simulink model "PlantaMalhaExterna"  (R2021a)
settings: Solver=VariableStepAuto  StartTime=0.0  StopTime=10.0  RelTol=1e-3
libraries: pid_lib x1
settings Model: Creator=lucas  LastModifiedBy=lucas

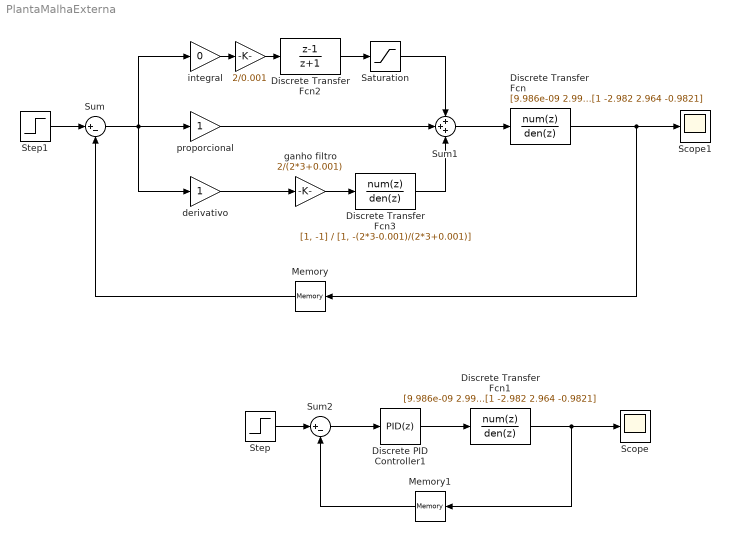
== system PlantaMalhaExterna ==
  " " : Gain  Gain=2/0.001
  Discrete Transfer Fcn : DiscreteTransferFcn  Numerator=[9.986e-09 2.996e-08 2.996e-08 9.986e-09]  Denominator=[1 -2.982 2.964 -0.9821]  SampleTime=0.001
  Discrete Transfer Fcn1 : DiscreteTransferFcn  Numerator=[9.986e-09 2.996e-08 2.996e-08 9.986e-09]  Denominator=[1 -2.982 2.964 -0.9821]  SampleTime=0.001
  Discrete Transfer Fcn2 : DiscreteTransferFcn  Numerator=[1, -1]  Denominator=[1, 1]
  Discrete Transfer Fcn3 : DiscreteTransferFcn  Numerator=[1, -1]  Denominator=[1, -(2*3-0.001)/(2*3+0.001)]  SampleTime=0.001
  Discrete PID Controller1 : pid_lib/PID Controller  Controller=PID  Form=Parallel  TimeDomain=Discrete-time  UseExternalTs=off  SampleTime=0.001  IntegratorMethod=Forward Euler  FilterMethod=Forward Euler  ControllerParametersSource=internal  P=200  I=0  D=8  UseFilter=on  N=1.824  TunerSelectOption=Transfer Function Based (PID Tuner App)  InitialConditionSource=internal  InitialConditionForIntegrator=0  InitialConditionForFilter=0  DifferentiatorICPrevScaledInput=0  ExternalReset=none  TrackingMode=off  Kt=1  LimitOutput=off  SatLimitsSource=internal  UpperSaturationLimit=inf  LowerSaturationLimit=-inf  LinearizeAsGain=off  AntiWindupMode=none  Kb=1  POutMin=[]  POutMax=[]  IOutMin=[]  IOutMax=[]  DOutMin=[]  DOutMax=[]  NOutMin=[]  NOutMax=[]  SumOutMin=[]  SumOutMax=[]  SaturationOutMin=[]  SaturationOutMax=[]  PParamMin=[]  PParamMax=[]  IParamMin=[]  IParamMax=[]  DParamMin=[]  DParamMax=[]  NParamMin=[]  NParamMax=[]  KbParamMin=[]  KbParamMax=[]  KtParamMin=[]  KtParamMax=[]  KbOutMin=[]  KbOutMax=[]  KtOutMin=[]  KtOutMax=[]  IntegratorOutMin=[]  IntegratorOutMax=[]  FilterOutMin=[]  FilterOutMax=[]  SumI1OutMin=[]  SumI1OutMax=[]  SumI2OutMin=[]  SumI2OutMax=[]  SumI3OutMin=[]  SumI3OutMax=[]  SumI4OutMin=[]  SumI4OutMax=[]  SumDOutMin=[]  SumDOutMax=[]  DifferentiatorOutMin=[]  DifferentiatorOutMax=[]  FilterDiffOutCoefMin=[]  FilterDiffOutCoefMax=[]  ReciprocalOutMin=[]  ReciprocalOutMax=[]  SumDenOutMin=[]  SumDenOutMax=[]  SumNumOutMin=[]  SumNumOutMax=[]  DivideOutMin=[]  DivideOutMax=[]  UdiffTsProdOutMin=[]  UdiffTsProdOutMax=[]  NTsProdOutMin=[]  NTsProdOutMax=[]  UintegralTsProdOutMin=[]  UintegralTsProdOutMax=[]  UngainTsProdOutMin=[]  UngainTsProdOutMax=[]  IntegratorContinuousStateAttributes=''  IntegratorStateMustResolveToSignalObject=off  IntegratorRTWStateStorageClass=Auto  FilterContinuousStateAttributes=''  FilterStateMustResolveToSignalObject=off  FilterRTWStateStorageClass=Auto  ParallelPVariant=InternalParameters  IdealPVariant=Disabled  IVariant=InternalParameters  DVariant=InternalParameters  IntegratorVariant=Discrete  SatVariant=Disabled  AWVariant=Passthrough  PCopyVariant=Disabled  TRVariant=Disabled  FdbkBlocksVariant=Forward  IdealPFdbkVariant=Disabled  SatFdbkVariant=Disabled  DerivativeFilterVariant=ForwardEulerFilter  NVariant=InternalParameters  NCopyVariant=Disabled  FilterICVariant=InternalICsFilter  IntegratorICVariant=InternalICs  ExternalResetVariant=Disabled  TRSumVariant=Passthrough  SumFdbkVariant=Disabled  SumVariant=Sum_PID  TsampFilterVariant=InternalTs  TsampNgainVariant=Passthrough  TsampIntegralVariant=Passthrough  ExternalSaturationOutDataTypeStr=Inherit: Same as second input
  Memory : Memory
  Memory1 : Memory
  Saturation : Saturate  UpperLimit=4095  LowerLimit=0
  Scope : Scope
  Scope1 : Scope
  Step : Step  Time=0  After=0.3  SampleTime=0.001
  Step1 : Step  Time=0  After=0.3  SampleTime=0.001
  Sum : Sum  Inputs=|+-
  Sum1 : Sum  Inputs=+++
  Sum2 : Sum  Inputs=|+-
  derivativo : Gain
  ganho filtro : Gain  Gain=2/(2*3+0.001)
  integral : Gain  Gain=0
  proporcional : Gain
  wires:
  Saturation/1 -> Sum1/1
  proporcional/1 -> Sum1/2
  Sum1/1 -> Discrete Transfer Fcn/1
  Discrete Transfer Fcn/1 -> Scope1/1, Memory/1
  Memory/1 -> Sum/2
  Sum/1 -> derivativo/1, integral/1, proporcional/1
  Discrete PID Controller1/1 -> Discrete Transfer Fcn1/1
  Memory1/1 -> Sum2/2
  Sum2/1 -> Discrete PID Controller1/1
  Discrete Transfer Fcn1/1 -> Scope/1, Memory1/1
  Step/1 -> Sum2/1
  Discrete Transfer Fcn3/1 -> Sum1/3
  Step1/1 -> Sum/1
  integral/1 -> " "/1
  " "/1 -> Discrete Transfer Fcn2/1
  Discrete Transfer Fcn2/1 -> Saturation/1
  derivativo/1 -> ganho filtro/1
  ganho filtro/1 -> Discrete Transfer Fcn3/1
